simulink model "second_order_sine_sweep"  (R2024b)
settings: Solver=ode8  StartTime=0.0  StopTime=6  FixedStep=0.0001  RelTol=1e-3
libraries: aerolibactuator x2, dspsrcs4 x1
settings Model: Creator=jonno  LastModifiedBy=jonno

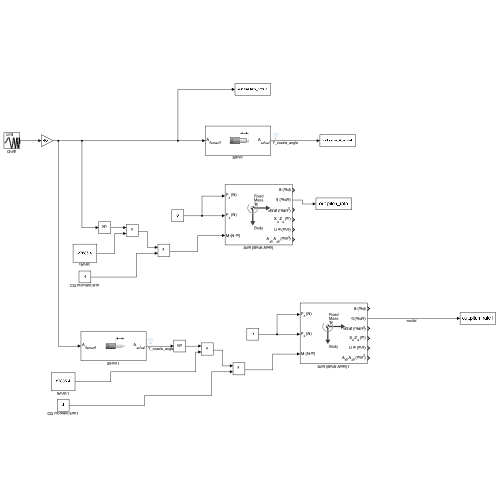
[thumbnail: Simulink's stored preview of the top-level diagram]
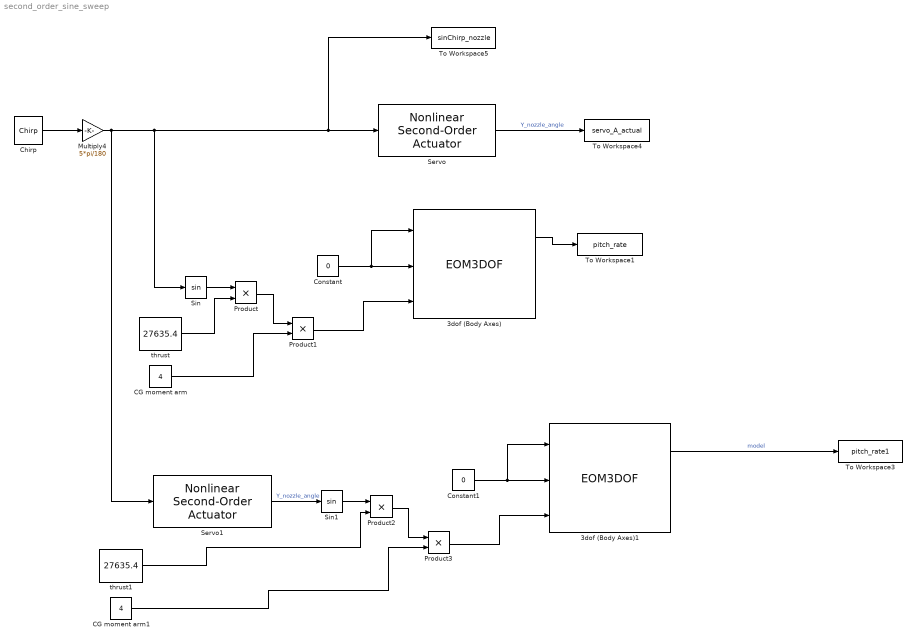
== system second_order_sine_sweep ==
  3dof (Body Axes) : EOM3DOF  v_ini=0  mass=974  Iyy=9470  g=0
  3dof (Body Axes)1 : EOM3DOF  v_ini=0  mass=974  Iyy=9470  g=0
  CG moment arm : Constant  Value=4
  CG moment arm1 : Constant  Value=4
  Chirp : dspsrcs4/Chirp  sweep=Logarithmic  mode=Unidirectional  f0=0.1  f1=100  t1=30  Tsweep=30  phase=0  Ts=0.0001  spf=1  datatype=double  OutputFrames=off
  Constant : Constant  Value=0
  Constant1 : Constant  Value=0
  Multiply4 : Gain  Gain=5*pi/180
  Product{,1..3} (4 alike) : Product
  Servo : aerolibactuator/Nonlinear Second-Order Actuator  wn_fin=95  z_fin=0.7  fin_max=10*pi/180  fin_min=-10*pi/180  fin_maxrate=(500*pi/180)  fin_act_0=0  fin_act_vel=0
  Servo1 : aerolibactuator/Nonlinear Second-Order Actuator  wn_fin=95  z_fin=0.7  fin_max=10*pi/180  fin_min=-10*pi/180  fin_maxrate=(500*pi/180)  fin_act_0=0  fin_act_vel=0
  Sin : Trigonometry
  Sin1 : Trigonometry
  To Workspace1 : ToWorkspace  VariableName=pitch_rate  SaveFormat=Timeseries  SampleTime=-1
  To Workspace3 : ToWorkspace  VariableName=pitch_rate1  SaveFormat=Timeseries  SampleTime=-1
  To Workspace4 : ToWorkspace  VariableName=servo_A_actual  SaveFormat=Timeseries  SampleTime=-1
  To Workspace5 : ToWorkspace  VariableName=sinChirp_nozzle  SaveFormat=Timeseries  SampleTime=-1
  thrust : Constant  Value=27635.4
  thrust1 : Constant  Value=27635.4
  wires:
  Chirp/1 -> Multiply4/1
  Servo/1 -> To Workspace4/1  "Y_nozzle_angle"
  Constant/1 -> 3dof (Body Axes)/1, 3dof (Body Axes)/2
  thrust/1 -> Product/2
  Sin/1 -> Product/1
  Product/1 -> Product1/1
  CG moment arm/1 -> Product1/2
  Product1/1 -> 3dof (Body Axes)/3
  3dof (Body Axes)/2 -> To Workspace1/1
  Product3/1 -> 3dof (Body Axes)1/3
  thrust1/1 -> Product2/2
  Product2/1 -> Product3/1
  3dof (Body Axes)1/2 -> To Workspace3/1  "model"
  Constant1/1 -> 3dof (Body Axes)1/1, 3dof (Body Axes)1/2
  Multiply4/1 -> Servo1/1, To Workspace5/1, Servo/1, Sin/1
  Sin1/1 -> Product2/1
  CG moment arm1/1 -> Product3/2
  Servo1/1 -> Sin1/1  "Y_nozzle_angle"
